simulink model "P4"  (R2023b)
settings: Solver=VariableStepAuto  StartTime=0.0  StopTime=10.0  MaxStep=0.001  RelTol=1e-3
values from neighbouring files (symbols this model uses):
  k = 100    [MR.m]    (also in P4parametros.m)
  m = 10    [MR.m]    (also in P4parametros.m)
settings Model: Creator=aquet  LastModifiedBy=aquet

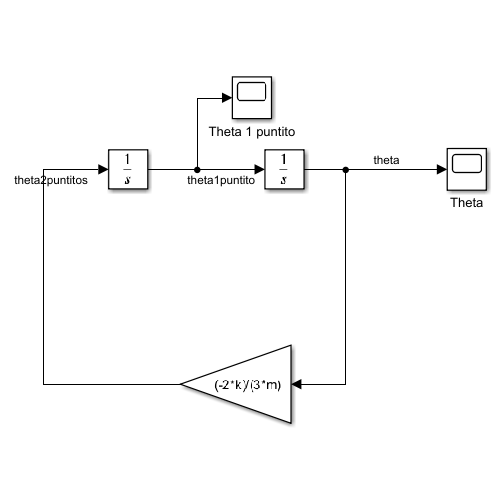
[thumbnail: Simulink's stored preview of the top-level diagram]
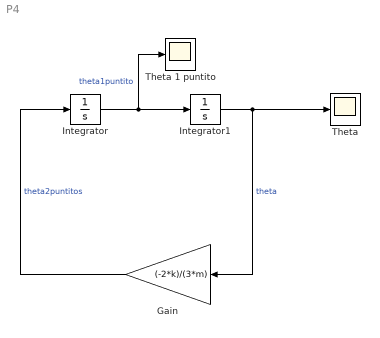
== system P4 ==
  Gain : Gain  Gain=(-2*k)/(3*m)
  Integrator : Integrator  InitialCondition=2
  Integrator1 : Integrator
  Theta : Scope
  Theta 1 puntito : Scope
  wires:
  Integrator/1 -> Theta 1 puntito/1, Integrator1/1  "theta1puntito"
  Gain/1 -> Integrator/1  "theta2puntitos"
  Integrator1/1 -> Theta/1, Gain/1  "theta"
